simulink model "hw2_1_d_sl"  (R2024a)
settings: Solver=VariableStepAuto  StartTime=0.0  StopTime=10.0  RelTol=1e-3
settings Model: Creator=CDSL-2  LastModifiedBy=CDSL-2

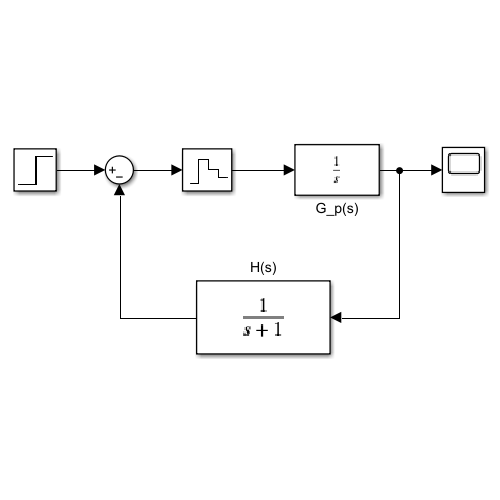
[thumbnail: Simulink's stored preview of the top-level diagram]
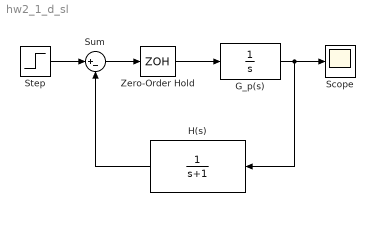
== system hw2_1_d_sl ==
  G_p(s) : TransferFcn  Denominator=[1 0]
  H(s) : TransferFcn  Denominator=[1 1]
  Scope : Scope
  Step : Step  SampleTime=0
  Sum : Sum  Inputs=|+-
  Zero-Order Hold : ZeroOrderHold  SampleTime=0.2
  wires:
  Zero-Order Hold/1 -> G_p(s)/1
  G_p(s)/1 -> Scope/1, H(s)/1
  H(s)/1 -> Sum/2
  Step/1 -> Sum/1
  Sum/1 -> Zero-Order Hold/1
